simulink model "Tesis1"  (Simulink 6.5)
settings: Solver=ode23t  StartTime=0.0  StopTime=1.4  RelTol=1e-6
undefined symbols (not defined in the file): powergui
libraries: powerlib x6, powerlib_extras x3
settings Model: Creator=RS  LastModifiedBy=PC_0
settings SolverCC: SolverResetMethod=Robust

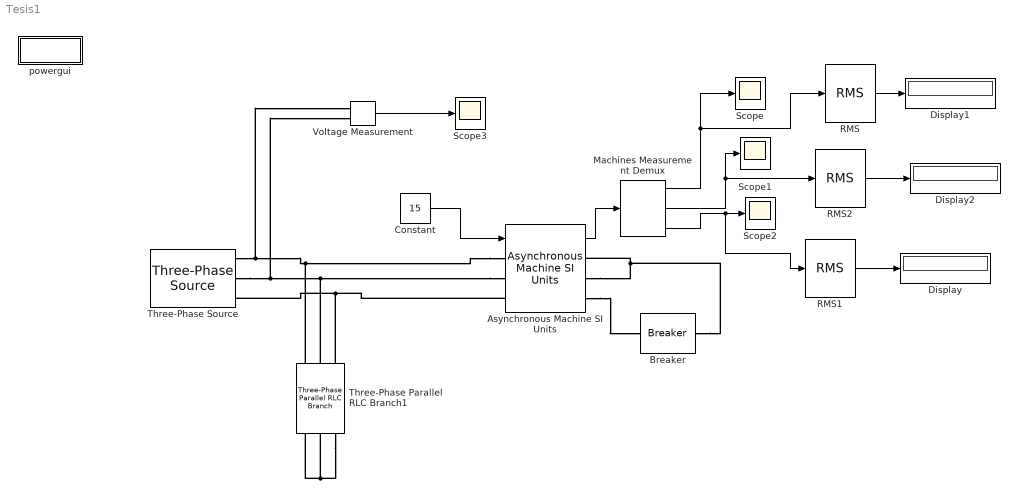
== system Tesis1 ==
  Asynchronous Machine SI Units : powerlib/Machines/Asynchronous Machine SI Units  DialogController=PMDialogs.PMDefaultMaskDlg  SystemSampleTime=-1  PresetModel=No  MechanicalLoad=Torque Tm  ShowDetailedParameters=on  RotorType=Wound  ReferenceFrame=Stationary  NominalParameters="[6.5*746    380   50]"  Stator="[0.63   0.00496]"  Rotor="[1.094   0.00496]"  Lm=0.105  Mechanical=[0.05 0.005752 2]  PolePairs=2  InitialConditions="[ 1,0   0,0,0   0,0,0 ]"  Units=1  LoadFlowParameters=0  SimulateSaturation=off  Saturation=[9.9249,19.6672,38.0377,51.3988,69.2824,105.1337,152.5532,214.2421,303.1917;230, 322, 414, 460, 506, 552, 598, 644, 690]
  Breaker : powerlib/Elements/Breaker  DialogController=PMDialogs.PMDefaultMaskDlg  SystemSampleTime=-1  BreakerResistance=0.00001  InitialState=1  SnubberResistance=1e6  SnubberCapacitance=inf  SwitchingTimes=0.6  External=off  Measurements=None  MoreParameters=off  NoBreakLoop=off
  Constant : Constant  Value=15  OutDataType=sfix(16)  ConRadixGroup=Use specified scaling  OutScaling=2^0  SampleTime=inf  FramePeriod=inf
  Display : Display
  Display1 : Display
  Display2 : Display
  Machines Measurement Demux : powerlib/Machines/Machines Measurement Demux  DialogController=PMDialogs.PMDefaultMaskDlg  SystemSampleTime=-1  machType=Asynchronous  ssm1=on  ssm2=on  ssm3=on  ssm4=on  ssm5=on  ssm6=on  sm1=off  sm2=off  sm3=off  sm4=off  sm5=off  sm6=off  sm7=off  sm8=on  sm9=off  sm10=off  sm11=off  sm115=off  sm12=off  sm13=off  sm14=off  asm1=off  asm2=off  asm3=off  asm4=off  asm5=on  asm6=off  asm7=off  asm8=off  asm9=on  asm10=on  asm11=off  pmsm1=on  pmsm2=on  pmsm3=on  pmsm4=off  pmsm5=on  pmsm6=on  pmsm7=on  lastType=1
  RMS : powerlib_extras/Measurements/RMS  DialogController=PMDialogs.PMDefaultMaskDlg  SystemSampleTime=-1  f1=50
  RMS1 : powerlib_extras/Measurements/RMS  DialogController=PMDialogs.PMDefaultMaskDlg  SystemSampleTime=-1  f1=50
  RMS2 : powerlib_extras/Measurements/RMS  DialogController=PMDialogs.PMDefaultMaskDlg  SystemSampleTime=-1  f1=50
  Scope{,1..3} (4 alike) : Scope
      Scope settings: MaxDataPoints=10000000  SampleInput=on  SampleTime=10e-6
      Scope1 settings: MaxDataPoints=10000000  SampleInput=on  SampleTime=10e-6
      Scope2 settings: TimeRange=1  YMin=10.8893  YMax=10.893  SaveName=ScopeData2  MaxDataPoints=10000000  SampleInput=on  SampleTime=10e-6
      Scope3 settings: SaveName=ScopeData3  MaxDataPoints=10000000  SampleInput=on  SampleTime=10e-6
  Three-Phase Parallel RLC Branch1 : powerlib/Elements/Three-Phase Parallel RLC Branch  Orientation=up  DialogController=PMDialogs.PMDefaultMaskDlg  PhysicalDomain=powersysdomain  SubClassName=unknown  LeftPortType=p1  RightPortType=p1  LConnTagsString=A|B|C  RConnTagsString=A|B|C  BranchType=R  Resistance=1000000  Inductance=1e-3  Capacitance=90e-6  Measurements=None
  Three-Phase Source : powerlib/Electrical Sources/Three-Phase Source  DialogController=PMDialogs.PMDefaultMaskDlg  SystemSampleTime=-1  Voltage=380  PhaseAngle=0  Frequency=50  InternalConnection=Yg  SpecifyImpedance=off  Resistance=0.0001  Inductance=0.0001  ShortCircuitLevel=100e6  BaseVoltage=25e3  XRratio=7
  Voltage Measurement : powerlib/Measurements/Voltage Measurement  DialogController=PMDialogs.PMDefaultMaskDlg  SystemSampleTime=-1  PhasorSimulation=off  OutputType=Complex  PSBequivalent=0
  powergui : Subsystem  AncestorBlock=powerlib/powergui  InitFcn=powergui( 'InitFcn_Callback' , gcb , 0 , [ ] );  mask(PSB option menu block){SimulationMode=Continuous, SampleTime=50e-6, echomessages=on, RestoreLinks=warning, x0status=blocks, Frange=[0:2:500], Ylog=off, Xlog=on, ShowGrid=off, save=off, variable=ZData, structure=ScopeData, ZoomFFT=off, StartTime=1, cycles=12, DisplayStyle=2, fundamental=50, FreqAxis=off, MaxFrequency=500, frequencyindice=50, frequencyindicesteady=1, RmsSteady=1, display=off, Ts=0, frequency=60, methode=off, HookPort=off, Interpol=off}
      mask prompts: SimulationMode "Simulation mode"; SampleTime "Sample time Ts (when simulation mode is Discrete) (s)"; echomessages "Echo  Messages"; RestoreLinks "Restore disabled links"; x0status "Initial electrical states status"; Frange "Impedance tool: Frequency Range"; Ylog "Impedance tool: Log impedance"; Xlog "Impedance tool: log Frequency"; ShowGrid "Impedance tool: grid"; save "Impedance tool: Save Data To Workspace"; variable "Impedance tool: Variable Name"; structure "Structure Name (PSBFFTSCOPE)"; ZoomFFT "ZoomFFT (PSBFFTSCOPE)"; StartTime "Start Time (PSBFFTSCOPE)"; cycles "Cycles (PSBFFTSCOPE)"; DisplayStyle "Display style (PSBFFTSCOPE)"; fundamental "Fundamental (PSBFFTSCOPE)"; FreqAxis "Frequency Axis (PSBFFTSCOPE)"; MaxFrequency "Max Frequency (PSBFFTSCOPE)"; frequencyindice "Load flow frequency (Hz)"; frequencyindicesteady "Frequency indice (STEADYSTATE)"; RmsSteady "RMS display (STEADYSTATE)"; display "Display Results"; Ts "OBSOLETE 1"; frequency "Phasor frequency (Hz)"; methode "Phasor simulation"; HookPort "Hook port"; Interpol "Interpolate"
      mask init:
      | powerlibroot = which('powersysdomain');
      | PSBroot = powerlibroot(1:end-16);
      | %
      | switch SimulationMode
      | 	case 1
      | 		message=sprintf('Continuous');
      | 	case 2
      |         SampleTimeeval=evalin('base',SampleTime,'NaN');
      |         if isnan(SampleTimeeval)
      |             message=sprintf('Warning !!,\nUndefined sample time');
      |         else
      |             message=sprintf('Discrete,\nTs = %.4g s.',SampleTimeeval);
      |         end
      | 	case 3
      | 		message=sprintf('Phasors');
      | end
      | if strcmp(bdroot,'powerlib')
      |   message='powergui';
      | end
      | power_initmask();
      settings: CopyFcn=powergui( 'Copy_Callback' , gcb , 0 , [ ] );  ModelCloseFcn=powergui( 'CloseButton_Callback' , gcb , [ ] , [ ] );  PreSaveFcn=powergui( 'CloseButton_Callback' , gcb , [ ] , [ ] );  NameChangeFcn=powergui( 'NameChangeFcn_Callback' , gcb , 0 , [ ] );
      settings: DeleteFcn=|
      | powergui( 'Copy_Callback' , gcb , 1 , [ ] );
      | powergui( 'CloseButton_Callback' , gcb , [ ] , [ ] );
      settings: OpenFcn=|
      | if (power_openblockproxy ('secondary'))
      | powergui(gcb,'PM')
      | end;
      mask Help: web(psbhelp)
      mask StyleString: popup(Continuous|Discrete|Phasor),edit,checkbox,popup(yes|warning|no),popup(blocks|steady|zero),edit,checkbox,checkbox,checkbox,checkbox,edit,edit,checkbox,edit,edit,edit,edit,checkbox,edit,edit,edit,edit,checkbox,edit,edit,checkbox,checkbox,checkbox
      mask CallbackString: ||||||||||||||||||||||||||powergui('HookPort',[],[],gcb);|
      mask Display: disp(message)
  wires:
  Constant/1 -> Asynchronous Machine SI Units/1
  Asynchronous Machine SI Units/1 -> Machines Measurement Demux/1
  Machines Measurement Demux/3 -> Scope2/1, RMS1/1
  Machines Measurement Demux/2 -> RMS2/1, Scope1/1
  Machines Measurement Demux/1 -> Scope/1, RMS/1
  RMS/1 -> Display1/1
  Voltage Measurement/1 -> Scope3/1
  RMS1/1 -> Display/1
  RMS2/1 -> Display2/1
  connections:
  Asynchronous Machine SI Units/LConn1 -- Three-Phase Source/RConn1 -- Voltage Measurement/LConn1 -- Three-Phase Parallel RLC Branch1/RConn1
  Asynchronous Machine SI Units/LConn2 -- Three-Phase Source/RConn2 -- Voltage Measurement/LConn2 -- Three-Phase Parallel RLC Branch1/RConn2
  Three-Phase Parallel RLC Branch1/LConn3 -- Three-Phase Parallel RLC Branch1/LConn1 -- Three-Phase Parallel RLC Branch1/LConn2
  Asynchronous Machine SI Units/RConn2 -- Asynchronous Machine SI Units/RConn1 -- Breaker/RConn1
  Asynchronous Machine SI Units/RConn3 -- Breaker/LConn1
  Asynchronous Machine SI Units/LConn3 -- Three-Phase Source/RConn3 -- Three-Phase Parallel RLC Branch1/RConn3

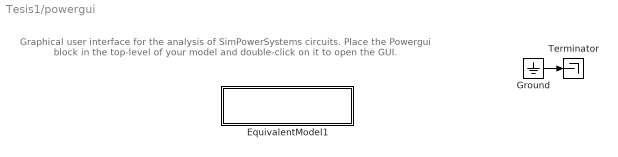
== system Tesis1/powergui ==
  note: Graphical user interface for the analysis of  SimPowerSystems circuits.
      | Place the Powergui block in the top-level of your model and double-click
      | on it to open the GUI.
  EquivalentModel1 : Subsystem
      mask init:
      | SPS = get_param(gcbh,'UserData');
      | if isempty(SPS)
      |     A=0;
      |     B=0;
      |     C=0;
      |     D=0;
      |     x0=0;
      |     SwitchResistance=1;
      |     SwitchType=1;
      |     SwitchGateInitialValue=1;
      |     OutputsToResetToZero=1;
      | else
      | 	A=SPS.A;
      |     B=SPS.B;
      |     C=SPS.C;
      |     D=SPS.D;
      |     x0=SPS.x0;
      |     SwitchResistance=SPS.SwitchResistance;
      |     SwitchType=SPS.SwitchType;
      |     SwitchGateInitialValue=SPS.SwitchGateInitialValue;
      |     OutputsToResetToZero=SPS.YSwitchCurrent;
      | end
      mask Display:
      | color('blue')
      | disp('EQUIVALENT CIRCUIT')
  Ground : Ground
  Terminator : Terminator
  wires:
  Ground/1 -> Terminator/1

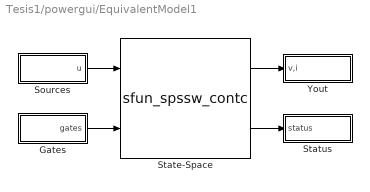
== system Tesis1/powergui/EquivalentModel1 ==
  Gates : Subsystem
  Sources : Subsystem
  State-Space : S-Function  FunctionName=sfun_spssw_contc  Parameters=A, B, C, D, x0, SwitchResistance ,SwitchType, SwitchGateInitialValue, OutputsToResetToZero
  Status : Subsystem
  Yout : Subsystem
  wires:
  Gates/1(gates) -> State-Space/2
  Sources/1(u) -> State-Space/1
  State-Space/2 -> Status/1(status)
  State-Space/1 -> Yout/1(v,i)

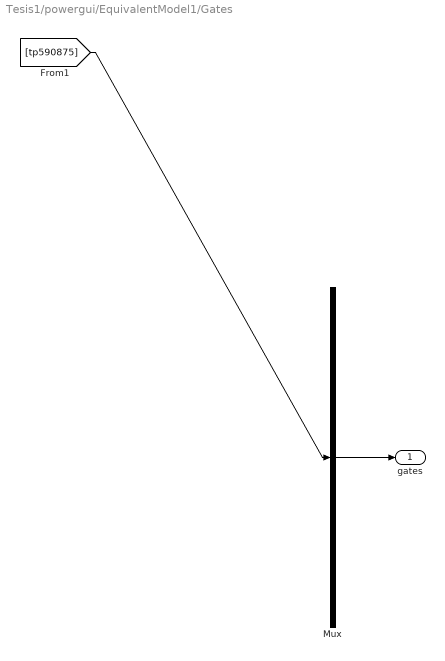
== system Tesis1/powergui/EquivalentModel1/Gates ==
  Mux : Mux  Inputs=1
  gates : Outport
  wires:
  Mux/1 -> gates/1
  [tp590875] -> Mux/1

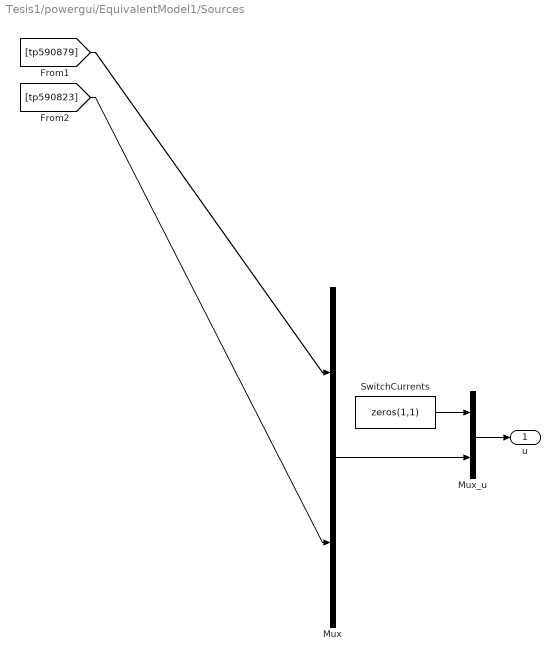
== system Tesis1/powergui/EquivalentModel1/Sources ==
  Mux : Mux  Inputs=[4 3]
  Mux_u : Mux  Inputs=[1 7]
  SwitchCurrents : Constant  Value=zeros(1,1)  OutDataType=sfix(16)  ConRadixGroup=Use specified scaling  OutScaling=2^0  SampleTime=inf  FramePeriod=inf
  u : Outport
  wires:
  Mux/1 -> Mux_u/2
  SwitchCurrents/1 -> Mux_u/1
  Mux_u/1 -> u/1
  [tp590879] -> Mux/1
  [tp590823] -> Mux/2

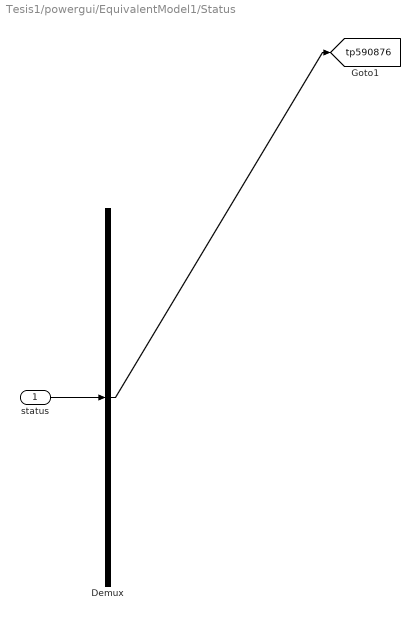
== system Tesis1/powergui/EquivalentModel1/Status ==
  status : Inport
  Demux : Demux  Outputs=1
  tag scope: tp590876=global
  wires:
  status/1 -> Demux/1
  Demux/1 -> [tp590876]

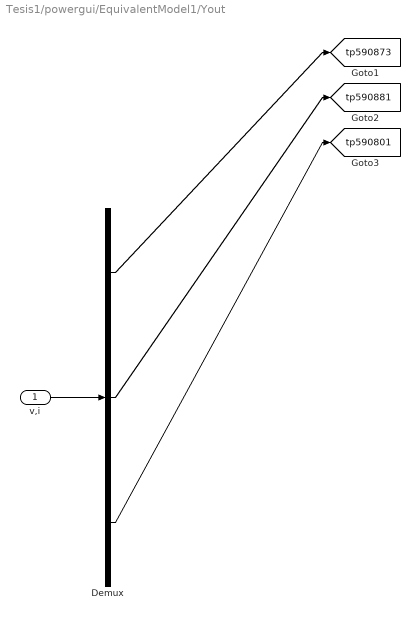
== system Tesis1/powergui/EquivalentModel1/Yout ==
  v,i : Inport
  Demux : Demux  Outputs=[1 4 1]
  tag scope: tp590801=global, tp590873=global, tp590881=global
  wires:
  v,i/1 -> Demux/1
  Demux/1 -> [tp590873]
  Demux/2 -> [tp590881]
  Demux/3 -> [tp590801]
